simulink library "relay_housing_lib"  (Simulink 8.1)
settings: Solver=ode45  StartTime=0.0  StopTime=10.0  RelTol=1e-3
undefined symbols (not defined in the file): F0, F1, F2, F3, F4, Ts
libraries: relay_modbus_lib x137, rtio_generic_modbus x69, rtlab x10, simulink_extras x10, simulink x6, RMS_lib x4, relay_PLL_lib x3, powerlib_extras x2, relay_ANSI_functions_lib x2, relay_PQSPF_lib x1, powerlib_meascontrol x1, relay_mgc_cmd_lib x1
(part 3 of 3)

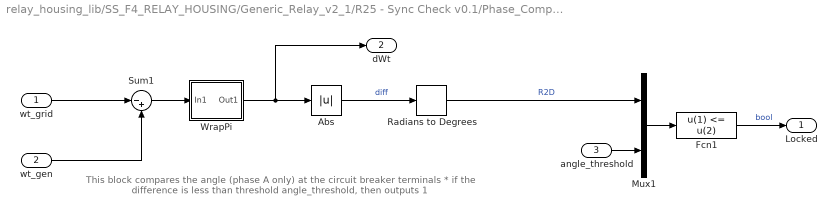
== system relay_housing_lib/SS_F4_RELAY_HOUSING/Generic_Relay_v2_1/R25 - Sync Check v0.1/Phase_Comparator ==
  note: This block compares the angle (phase A only) at the circuit breaker terminals
      | * if the difference is less than threshold angle_threshold, then outputs 1
  wt_grid : Inport
  wt_gen : Inport  Port=2
  angle_threshold : Inport  Port=3
  Abs : Abs
  Fcn1 : Fcn  Expr=u(1) <= u(2)  SampleTime=Ts
  Mux1 : Mux  Inputs=2
  Radians to Degrees : simulink_extras/Transformations/Radians to Degrees
  Sum1 : Sum  Inputs=|-+
  WrapPi : Subsystem
  Locked : Outport
  dWt : Outport  Port=2
  wires:
  Abs/1 -> Radians to Degrees/1  "diff"
  Fcn1/1 -> Locked/1  "bool"
  angle_threshold/1 -> Mux1/2
  Mux1/1 -> Fcn1/1
  Radians to Degrees/1 -> Mux1/1  "R2D"
  wt_gen/1 -> Sum1/2
  wt_grid/1 -> Sum1/1
  Sum1/1 -> WrapPi/1(In1)
  WrapPi/1(Out1) -> dWt/1, Abs/1

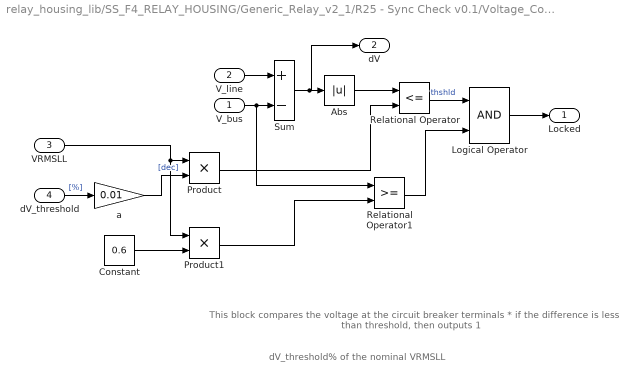
== system relay_housing_lib/SS_F4_RELAY_HOUSING/Generic_Relay_v2_1/R25 - Sync Check v0.1/Voltage_Comparator ==
  note: dV_threshold% of the nominal VRMSLL
  note: This block compares the voltage at the circuit breaker terminals
      | * if the difference is less than threshold, then outputs 1
  V_bus : Inport
  V_line : Inport  Port=2
  VRMSLL : Inport  Port=3
  dV_threshold : Inport  Port=4
  Abs : Abs
  Constant : Constant  Value=0.6
  Logical Operator : Logic  AllPortsSameDT=off  OutDataTypeStr=boolean
  Product : Product
  Product1 : Product
  Relational Operator : RelationalOperator  Operator=<=  OutDataTypeStr=boolean
  Relational Operator1 : RelationalOperator  OutDataTypeStr=boolean
  Sum : Sum  Inputs=+-
  a : Gain  Gain=0.01
  Locked : Outport
  dV : Outport  Port=2
  wires:
  Relational Operator1/1 -> Logical Operator/2
  Abs/1 -> Relational Operator/1
  Product1/1 -> Relational Operator1/2
  Constant/1 -> Product1/2
  Logical Operator/1 -> Locked/1
  a/1 -> Product/2  "[dec]"
  Relational Operator/1 -> Logical Operator/1  "thshld"
  V_line/1 -> Sum/1
  V_bus/1 -> Sum/2, Relational Operator1/1
  dV_threshold/1 -> a/1  "[%]"
  VRMSLL/1 -> Product/1, Product1/1
  Product/1 -> Relational Operator/2
  Sum/1 -> Abs/1, dV/1

== system relay_housing_lib/SS_F4_RELAY_HOUSING/Generic_Relay_v2_1/R25 - Sync Check v0.1/Phase_Comparator/WrapPi ==
  In1 : Inport
  Compare To Constant1 : simulink/Logic and Bit Operations/Compare To Constant  relop=<=  const=-pi  OutDataTypeStr=boolean
  Compare To Constant2 : simulink/Logic and Bit Operations/Compare To Constant  relop=>=  const=pi  OutDataTypeStr=boolean
  Gain1 : Gain  Gain=2*pi
  Gain2 : Gain  Gain=2*pi
  Sum : Sum  Inputs=++-
  Out1 : Outport
  wires:
  Sum/1 -> Out1/1
  Gain1/1 -> Sum/1
  Gain2/1 -> Sum/3
  In1/1 -> Compare To Constant2/1, Compare To Constant1/1, Sum/2
  Compare To Constant1/1 -> Gain1/1
  Compare To Constant2/1 -> Gain2/1

== matlab function SS_F4_RELAY_HOUSING/Generic_Relay_v2_1/R25 - Sync Check v0.1/deadbus fcn ==
  data: Vbus input double; y output double; Vline input double; VRMSLL input double
% Copyright (c) 2016 Massachusetts Institute of Technology
% Permission is hereby granted, free of charge, to any person obtaining a copy of this
% software and associated documentation files (the "Software"), to deal in the Software
% without restriction, including without limitation the rights to use, copy, modify,
% merge, publish, distribute, sublicense, and/or sell copies of the Software, and to
% permit persons to whom the Software is furnished to do so, subject to the following
% conditions:
%
%
% The above copyright notice and this permission notice shall be included in
% all copies or substantial portions of the Software.
%
% THE SOFTWARE IS PROVIDED "AS IS", WITHOUT WARRANTY OF ANY KIND, EXPRESS OR IMPLIED,
% INCLUDING BUT NOT LIMITED TO THE WARRANTIES OF MERCHANTABILITY, FITNESS FOR A
% PARTICULAR PURPOSE AND NONINFRINGEMENT. IN NO EVENT SHALL THE AUTHORS OR COPYRIGHT
% HOLDERS BE LIABLE FOR ANY CLAIM, DAMAGES OR OTHER LIABILITY, WHETHER IN AN ACTION
% OF CONTRACT, TORT OR OTHERWISE, ARISING FROM, OUT OF OR IN CONNECTION WITH THE
% SOFTWARE OR THE USE OR OTHER DEALINGS IN THE SOFTWARE.
%
%
%%

function y = fcn(Vbus, Vline, VRMSLL)
%#codegen
if isnan(Vbus)
    Vbus=0;
elseif isnan(Vline)
    Vline = 0;
end

% voltage threshold for deadbus
if VRMSLL > 520
    threshold = VRMSLL * 0.03; % @ 3%
else
    threshold = VRMSLL * 0.05; % @ 5%
end

% selecting 10V as the deadbus band - similar to SEL751
% threshold = 10;

% bounding open-circuit voltage at 120%
a = (Vbus>(VRMSLL*0.85)) && (Vbus<(VRMSLL*1.20)) && (Vline < threshold);
%b = (Vline>(VRMSLL*0.8)) && (Vline<(VRMSLL*1.20)) && (Vbus < threshold); -
% disabled for CB401 - voltage must be available on grid sim
% c = (Vline < threshold) && (Vbus < threshold);
y = a; %||b||c;
